simulink model "lab3_ss_srl"  (R2024b)
settings: Solver=ode45  StartTime=0.0  StopTime=sIn.simulation_time  RelTol=1e-3
undefined symbols (not defined in the file or in its folder): daq, DiscIntNeverNeededParam, drv, feedback, filt, gbox, mld, mot, rads2rpm, sens, sIn
libraries: simulink x1
settings Model: Creator=pries  LastModifiedBy=Nihal
settings DataIOCC: SaveOutput=off  SaveTime=off  ReturnWorkspaceOutputs=off

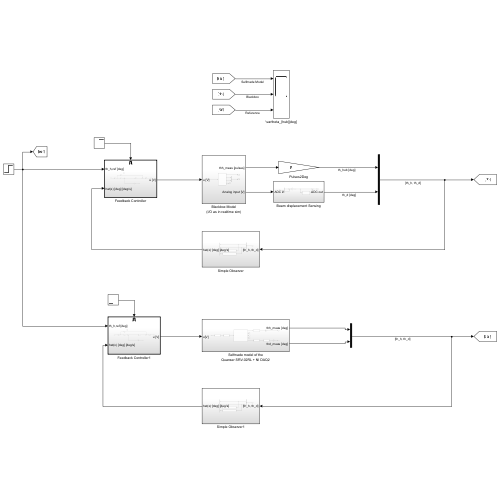
[thumbnail: Simulink's stored preview of the top-level diagram]
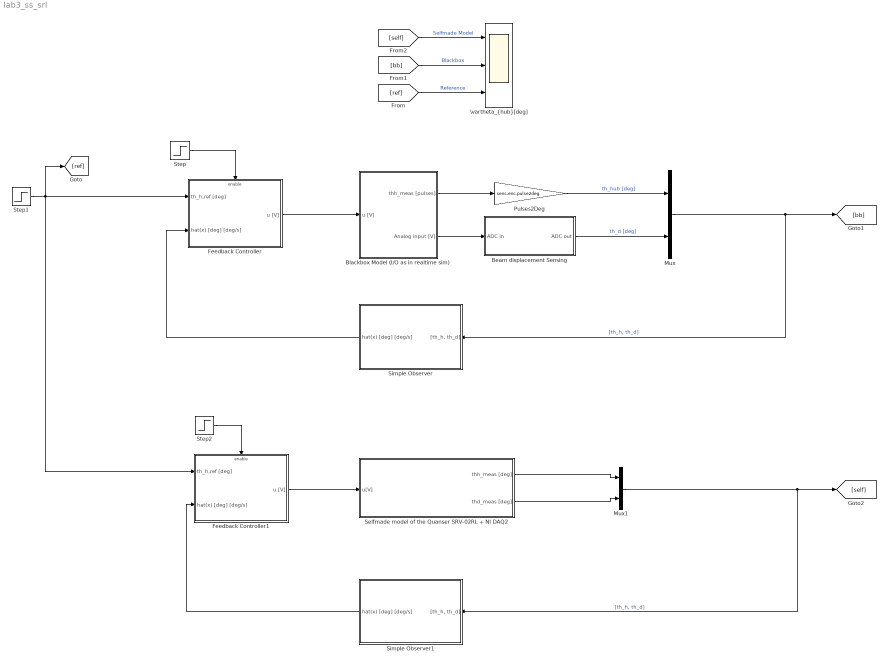
== system lab3_ss_srl ==
  Beam displacement Sensing : Subsystem
  Blackbox Model (I/O as in realtime sim) : Subsystem
  Feedback Controller : Subsystem
  Feedback Controller1 : Subsystem
  Mux : Mux  Inputs=2
  Mux1 : Mux  Inputs=2
  Pulses2Deg : Gain  Gain=sens.enc.pulse2deg
  Selfmade model of the Quanser SRV-02RL + NI DAQ2 : Subsystem
  Simple Observer : Subsystem
  Simple Observer1 : Subsystem
  Step : Step  Time=sIn.t1  SampleTime=0
  Step1 : Step  Time=sIn.t1  After=sIn.position  SampleTime=0
  Step2 : Step  Time=sIn.t1  SampleTime=0
  "\\vartheta_{hub}[deg]" : Scope  NumInputPorts=3
  wires:
  Pulses2Deg/1 -> Mux/1  "th_hub [deg]"
  Mux/1 -> [bb], Simple Observer/1("[th_h, th_d]")  "[th_h, th_d]"
  Simple Observer/1(hat(x) [deg] [deg/s]) -> Feedback Controller/2(hat(x) [deg] [deg/s])
  Blackbox Model (I/O as in realtime sim)/1(thh_meas [pulses]) -> Pulses2Deg/1
  Blackbox Model (I/O as in realtime sim)/2(Analog input [V]) -> Beam displacement Sensing/1(ADC in)
  Beam displacement Sensing/1(ADC out) -> Mux/2  "th_d [deg]"
  Step/1 -> Feedback Controller/Enable
  Feedback Controller/1(u [V]) -> Blackbox Model (I/O as in realtime sim)/1(u [V])
  Step1/1 -> Feedback Controller1/1(th_h,ref [deg]), Feedback Controller/1(th_h,ref [deg]), [ref]
  Simple Observer1/1(hat(x) [deg] [deg/s]) -> Feedback Controller1/2(hat(x) [deg] [deg/s])
  Mux1/1 -> Simple Observer1/1("[th_h, th_d]"), [self]  "[th_h, th_d]"
  [self] -> "\\vartheta_{hub}[deg]"/1  "Selfmade Model"
  [bb] -> "\\vartheta_{hub}[deg]"/2  "Blackbox"
  [ref] -> "\\vartheta_{hub}[deg]"/3  "Reference"
  Feedback Controller1/1(u [V]) -> Selfmade model of the Quanser SRV-02RL + NI DAQ2/1(u[V])
  Step2/1 -> Feedback Controller1/Enable
  Selfmade model of the Quanser SRV-02RL + NI DAQ2/1(thh_meas [deg]) -> Mux1/1
  Selfmade model of the Quanser SRV-02RL + NI DAQ2/2(thd_meas [deg]) -> Mux1/2

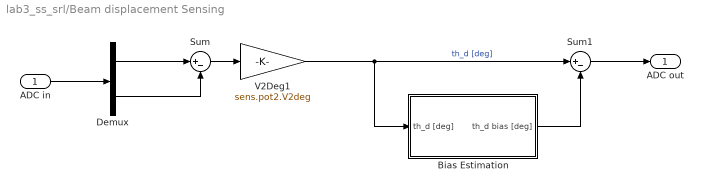
== system lab3_ss_srl/Beam displacement Sensing ==
  ADC in : Inport
  Bias Estimation : Subsystem
  Demux : Demux  Outputs=2
  Sum : Sum  Inputs=|+-
  Sum1 : Sum  Inputs=|+-
  V2Deg1 : Gain  Gain=sens.pot2.V2deg
  ADC out : Outport
  wires:
  Bias Estimation/1(th_d bias [deg]) -> Sum1/2
  ADC in/1 -> Demux/1
  V2Deg1/1 -> Bias Estimation/1(th_d [deg]), Sum1/1  "th_d [deg]"
  Sum/1 -> V2Deg1/1
  Demux/2 -> Sum/2
  Demux/1 -> Sum/1
  Sum1/1 -> ADC out/1

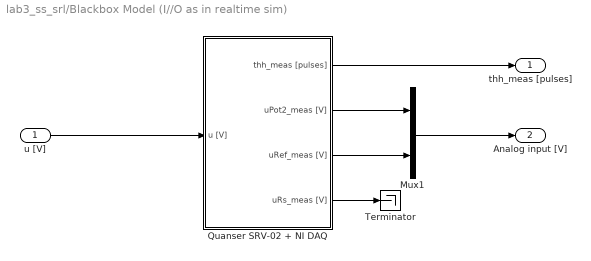
== system lab3_ss_srl/Blackbox Model (I//O as in realtime sim) ==
  u [V] : Inport
  Mux1 : Mux  Inputs=2
  Quanser SRV-02 + NI DAQ : Subsystem  mask(Quanser SRV-02 (with resonant load) + NI DAQ){Ts=0.001, fricType=Coulomb + viscous, lockShaft=off, beamInitPos=10}
      mask prompts: Ts "NI DAQ Sample Time:"; fricType "Friction model"; lockShaft "Lock motor shaft"; beamInitPos "Beam initial position [deg]:"
      mask help: Quanser SRV-02 (with resonant load) + NI DAQ model.
      mask init:
      | %%
      | % Riccardo Antonello (riccardo.antonello@unipd.it)
      | %
      | % April 28, 2020
      | %
      | % Dept. of Information Engineering, University of Padova
      | %
      | 
      | %%  Conversion gains
      | deg2rad = pi/180;                   %   [deg]   -> [rad]
      | rad2deg = 180/pi;                   %   [rad]   -> [deg]
      | 
      | 
      | %%  Sensors data
      | 
      | %   shunt resistor
      | sens.curr.Rs = 0.5;   
      | 
      | %   Hewlett-Packard HEDS-5540#A06 optical encoder
      | sens.enc.ppr = 500*4;                                                   %   pulses per rotation
      | sens.enc.pulse2deg = 360/sens.enc.ppr;                                  %   [pulses] -> [deg]
      | sens.enc.pulse2rad = 2*pi/sens.enc.ppr;                                 %   [pulses] -> [rad]
      | sens.enc.deg2pulse = sens.enc.ppr/360;                                  %   [deg] -> [pulses]
      | sens.enc.rad2pulse = sens.enc.ppr/2/pi;                                 %   [rad] -> [pulses]
      | 
      | %   potentiometer 2 (Spectrol 357-0-0-103) - installed on hub
      | sens.pot2.range.R      = 10e3;                                          %   ohmic value range 
      | sens.pot2.range.V      = 5;                                             %   voltage range
      | sens.pot2.range.th_deg = 340;                                           %   angle range [deg]
      | sens.pot2.range.th     = sens.pot2.range.th_deg * deg2rad;              %   angle range [rad]                           
      | sens.pot2.deg2V        = sens.pot2.range.V / sens.pot2.range.th_deg;    %   sensitivity [V/deg]
      | sens.pot2.rad2V        = sens.pot2.range.V / sens.pot2.range.th;        %   sensitivity [V/rad]
      | sens.pot2.V2deg        = 1/sens.pot2.deg2V;                             %   conversion gain [V] -> [deg]
      | sens.pot2.V2rad        = 1/sens.pot2.rad2V;                             %   conversion gain [V] -> [rad]
      | sens.pot2.noise.var    = 3.5e-7;                                        %   out noise variance [V^2]
      | 
      | 
      | %%  Data acquisition board (daq) data
      | 
      | %   NI PCI-6221 DAC data
      | daq.dac.bits = 16;                                  %   resolution (bits)
      | daq.dac.fs   = 10;                                  %   full scale 
      | daq.dac.q    = 2*daq.dac.fs/(2^daq.dac.bits-1);     %	quantization
      | 
      | %   NI PCI-6221 ADC data
      | daq.adc.bits = 16;                                  %   resolution (bits)
      | daq.adc.fs   = 10;                                  %   full scale (as set in SLDRT Analog Input block)
      | daq.adc.q    = 2*daq.adc.fs/(2^daq.adc.bits-1);     %   quantization   
      | 
      | 
      | %%  Set beam initial position
      | % SRV02Handle = find_system(gcb, ...
      | %     'LookUnderMasks', 'on', ...
      | %     'FindAll', 'on', ...
      | %     'FollowLinks', 'on', ...
      | %     'SearchDepth', '1', ...
      | %     'BlockType', 'ModelReference', ...
      | %     'Name', 'Quanser SRV-02');
      | %
      | % %get_param(SRV02Handle, 'InstanceParameters')
      | % InstanceParams = get_param(SRV02Handle, 'InstanceParameters');
      | % for k = 1:length(InstanceParams)
      | %     if strcmp(InstanceParams(k).Name, 'thb0')
      | %         if lockShaft
      | %             InstanceParams(k).Value = sprintf('%f', beamInitPos);
      | %         else
      | %             InstanceParams(k).Value = sprintf('%f', 0);    
      | %         end
      | %         set_param(SRV02Handle, 'InstanceParameters', InstanceParams);
      | %         break;
      | %     end
      | % end
      | 
      | if lockShaft
      |     thb0 = beamInitPos;
      | else
      |     thb0 = 0;    
      | end
      | 
      | 
      | %%  Mask initialization
      | if lockShaft
      |     
      |     %   find Inport handle
      |     InPortHandle = find_system(gcb, ...
      |         'LookUnderMasks', 'on', ...
      |         'FindAll', 'on', ...
      |         'FollowLinks', 'on', ...
      |         'SearchDepth', '1', ...
      |         'BlockType', 'Inport', ...
      |         'Name', 'u [V]');
      |     
      |     if ~isempty(InPortHandle)
      |     
      |         %   find DAC handle
      |         DACHandle = find_system(gcb, ...
      |             'LookUnderMasks', 'on', ...
      |             'FindAll', 'on', ...
      |             'FollowLinks', 'on', ...
      |             'SearchDepth', '1', ...
      |             'BlockType', 'SubSystem', ...
      |             'Name', 'DAC');  
      | 
      |         %   remove Inport output connection   
      |         InportConn = get_param(InPortHandle, 'PortConnectivity');
      |         delete_line(gcb, InportConn.Position);
      | 
      |         %   remove Inport block
      |         delete_block(InPortHandle);
      | 
      |         %   add Constant block
      |         ConstantHandle = add_block( ...
      |             'simulink/Sources/Constant', [gcb, '/u [V]'], ...
      |             'Position', [20   -37    50   -23], ...
      |             'Value', '0');
      | 
      |         %   connect Constant to DAC block
      |         DACPortHandles = get_param(DACHandle, 'PortHandles');
      |         ConstantPortHandles = get_param(ConstantHandle, 'PortHandles');
      |         add_line(gcb, ConstantPortHandles.Outport(1), DACPortHandles.Inport(1));
      |     
      |     end
      |     
      | else
      |     
      |     %   find Constant handle
      |     ConstantHandle = find_system(gcb, ...
      |         'LookUnderMasks', 'on', ...
      |         'FindAll', 'on', ...
      |         'FollowLinks', 'on', ...
      |         'SearchDepth', '1', ...
      |         'BlockType', 'Constant', ...
      |         'Name', 'u [V]');
      |     
      |     if ~isempty(ConstantHandle)
      |     
      |         %   find DAC handle
      |         DACHandle = find_system(gcb, ...
      |             'LookUnderMasks', 'on', ...
      |             'FindAll', 'on', ...
      |             'FollowLinks', 'on', ...
      |             'SearchDepth', '1', ...
      |             'BlockType', 'SubSystem', ...
      |             'Name', 'DAC');  
      |  
      |         %   remove Constant output connection   
      |         ConstantConn = get_param(ConstantHandle, 'PortConnectivity');
      |         delete_line(gcb, ConstantConn.Position);
      | 
      |         %   remove Inport block
      |         delete_block(ConstantHandle);   
      | 
      |         %   add Inport block
      |         InportHandle = add_block( ...
      |             'simulink/Sources/In1', [gcb, '/u [V]'], ...
      |             'Position', [20   -37    50   -23], ...
      |             'Port', '1');
      | 
      |         %   connect Constant to DAC block
      |         DACPortHandles = get_param(DACHandle, 'PortHandles');
      |         InportPortHandles = get_param(InportHandle, 'PortHandles');
      |         add_line(gcb, InportPortHandles.Outport(1), DACPortHandles.Inport(1));
      |     
      |      end
      |     
      | end
      mask Help:
      | Riccardo Antonello (antonello@dei.unipd.it)
      | 
      | April 28, 2020
      | 
      | Dept. of Information Engineering, University of Padova
      mask TypeOptions fricType: Coulomb + viscous | Karnopp
      mask Callback lockShaft:
      | %   get status of check box
      | lockShaft = get_param(gcb, 'lockShaft');
      | 
      | %   get current value of MaskVisibilities property
      | maskVisibilities = get_param(gcb, 'MaskVisibilities');
      | 
      | %   set visibility of the dialog box element
      | if strcmp(lockShaft, 'on')
      |     maskVisibilities{4} = 'on';
      | else
      |     maskVisibilities{4} = 'off';
      | end
      | 
      | % Set the 'MaskVisibilities' property for each parameter in mask
      | set_param( gcb, 'MaskVisibilities', maskVisibilities);
  Terminator : Terminator
  thh_meas [pulses] : Outport
  Analog input [V] : Outport  Port=2
  wires:
  Quanser SRV-02 + NI DAQ/1(thh_meas [pulses]) -> thh_meas [pulses]/1
  Quanser SRV-02 + NI DAQ/4(uRs_meas [V]) -> Terminator/1
  Mux1/1 -> Analog input [V]/1
  Quanser SRV-02 + NI DAQ/3(uRef_meas [V]) -> Mux1/2
  Quanser SRV-02 + NI DAQ/2(uPot2_meas [V]) -> Mux1/1
  u [V]/1 -> Quanser SRV-02 + NI DAQ/1(u [V])

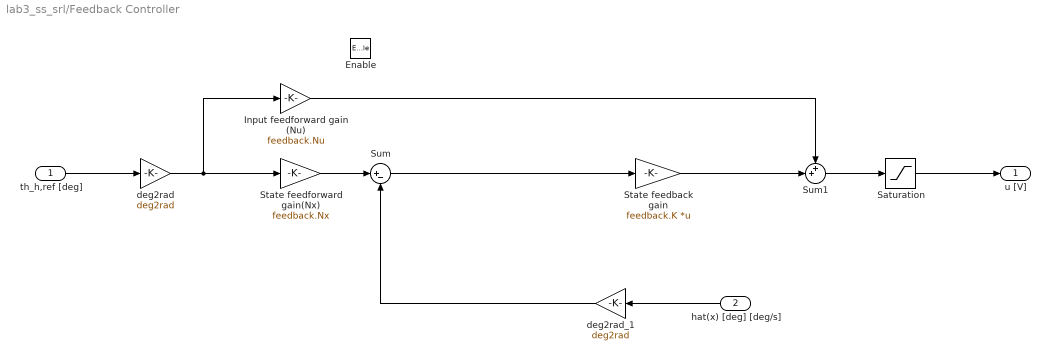
== system lab3_ss_srl/Feedback Controller ==
  th_h,ref [deg] : Inport
  hat(x) [deg] [deg/s] : Inport  Port=2
  Enable : EnablePort
  Input feedforward gain (Nu) : Gain  Gain=feedback.Nu
  Saturation : Saturate  UpperLimit=10  LowerLimit=-10
  State feedback gain : Gain  Gain=feedback.K  Multiplication=Matrix(K*u)
  State feedforward gain(Nx) : Gain  Gain=feedback.Nx
  Sum : Sum  Inputs=|+-
  Sum1 : Sum  Inputs=++|
  deg2rad : Gain  Gain=deg2rad
  deg2rad_1 : Gain  Gain=deg2rad
  u [V] : Outport
  wires:
  deg2rad_1/1 -> Sum/2
  Input feedforward gain (Nu)/1 -> Sum1/1
  State feedback gain/1 -> Sum1/2
  Sum1/1 -> Saturation/1
  Sum/1 -> State feedback gain/1
  Saturation/1 -> u [V]/1
  State feedforward gain(Nx)/1 -> Sum/1
  deg2rad/1 -> State feedforward gain(Nx)/1, Input feedforward gain (Nu)/1
  th_h,ref [deg]/1 -> deg2rad/1
  hat(x) [deg] [deg/s]/1 -> deg2rad_1/1

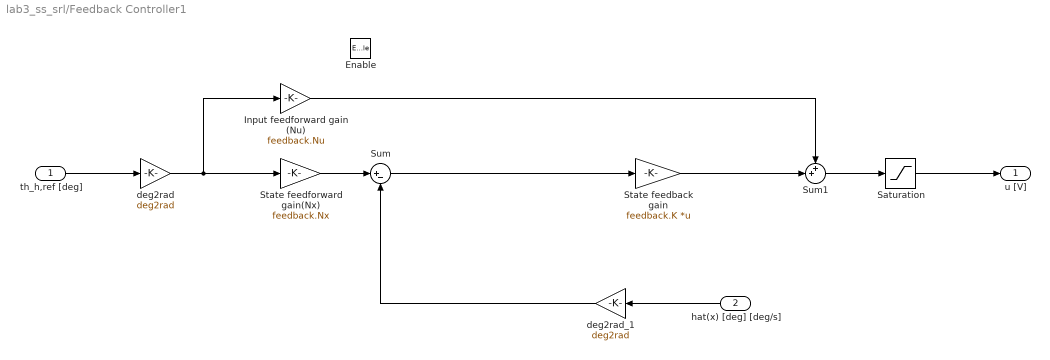
== system lab3_ss_srl/Feedback Controller1 ==
  th_h,ref [deg] : Inport
  hat(x) [deg] [deg/s] : Inport  Port=2
  Enable : EnablePort
  Input feedforward gain (Nu) : Gain  Gain=feedback.Nu
  Saturation : Saturate  UpperLimit=10  LowerLimit=-10
  State feedback gain : Gain  Gain=feedback.K  Multiplication=Matrix(K*u)
  State feedforward gain(Nx) : Gain  Gain=feedback.Nx
  Sum : Sum  Inputs=|+-
  Sum1 : Sum  Inputs=++|
  deg2rad : Gain  Gain=deg2rad
  deg2rad_1 : Gain  Gain=deg2rad
  u [V] : Outport
  wires:
  deg2rad_1/1 -> Sum/2
  Input feedforward gain (Nu)/1 -> Sum1/1
  State feedback gain/1 -> Sum1/2
  Sum1/1 -> Saturation/1
  Sum/1 -> State feedback gain/1
  Saturation/1 -> u [V]/1
  State feedforward gain(Nx)/1 -> Sum/1
  deg2rad/1 -> State feedforward gain(Nx)/1, Input feedforward gain (Nu)/1
  th_h,ref [deg]/1 -> deg2rad/1
  hat(x) [deg] [deg/s]/1 -> deg2rad_1/1

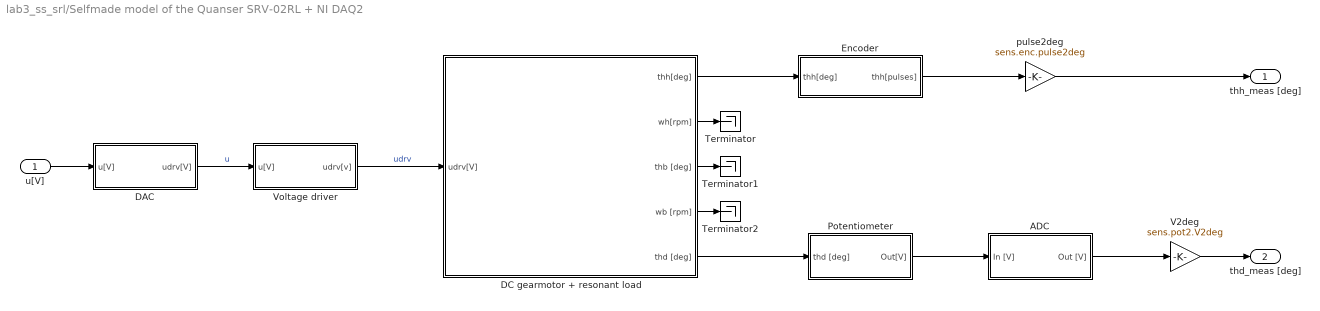
== system lab3_ss_srl/Selfmade model of the Quanser SRV-02RL + NI DAQ2 ==
  u[V] : Inport
  ADC : Subsystem
  DAC : Subsystem
  DC gearmotor + resonant load : Subsystem
  Encoder : Subsystem
  Potentiometer : Subsystem
  Terminator : Terminator
  Terminator1 : Terminator
  Terminator2 : Terminator
  V2deg : Gain  Gain=sens.pot2.V2deg
  Voltage driver : Subsystem
  pulse2deg : Gain  Gain=sens.enc.pulse2deg
  thh_meas [deg] : Outport
  thd_meas [deg] : Outport  Port=2
  wires:
  u[V]/1 -> DAC/1(u[V])
  DAC/1(udrv[V]) -> Voltage driver/1(u[V])  "u"
  Voltage driver/1(udrv[v]) -> DC gearmotor + resonant load/1(udrv[V])  "udrv"
  DC gearmotor + resonant load/1(thh[deg]) -> Encoder/1(thh[deg])
  Encoder/1(thh[pulses]) -> pulse2deg/1
  pulse2deg/1 -> thh_meas [deg]/1
  V2deg/1 -> thd_meas [deg]/1
  DC gearmotor + resonant load/5(thd [deg]) -> Potentiometer/1(thd [deg])
  DC gearmotor + resonant load/4(wb [rpm]) -> Terminator2/1
  DC gearmotor + resonant load/3(thb [deg]) -> Terminator1/1
  DC gearmotor + resonant load/2(wh[rpm]) -> Terminator/1
  Potentiometer/1(Out[V]) -> ADC/1(In [V])
  ADC/1(Out [V]) -> V2deg/1

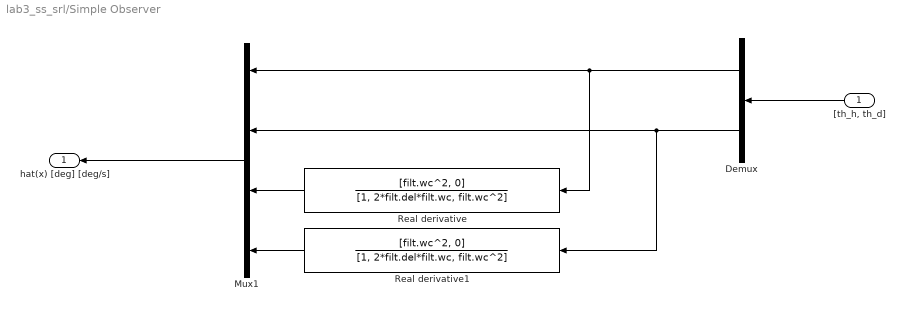
== system lab3_ss_srl/Simple Observer ==
  "[th_h, th_d]" : Inport
  Demux : Demux  Outputs=2
  Mux1 : Mux
  Real derivative : TransferFcn  Numerator=[filt.wc^2, 0]  Denominator=[1, 2*filt.del*filt.wc, filt.wc^2]
  Real derivative1 : TransferFcn  Numerator=[filt.wc^2, 0]  Denominator=[1, 2*filt.del*filt.wc, filt.wc^2]
  hat(x) [deg] [deg/s] : Outport
  wires:
  Demux/1 -> Mux1/1, Real derivative/1
  Mux1/1 -> hat(x) [deg] [deg/s]/1
  "[th_h, th_d]"/1 -> Demux/1
  Real derivative/1 -> Mux1/3
  Demux/2 -> Real derivative1/1, Mux1/2
  Real derivative1/1 -> Mux1/4

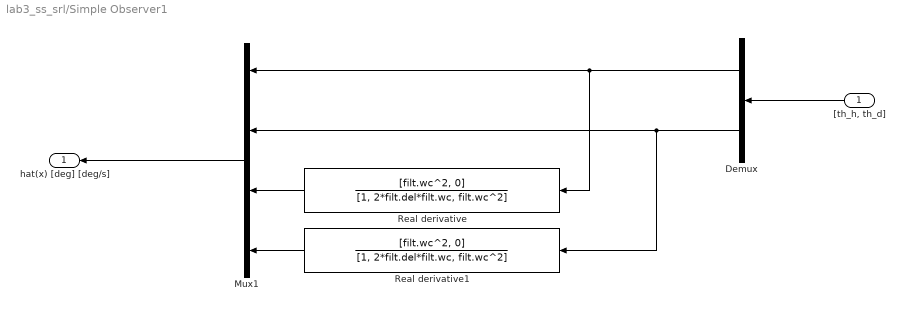
== system lab3_ss_srl/Simple Observer1 ==
  "[th_h, th_d]" : Inport
  Demux : Demux  Outputs=2
  Mux1 : Mux
  Real derivative : TransferFcn  Numerator=[filt.wc^2, 0]  Denominator=[1, 2*filt.del*filt.wc, filt.wc^2]
  Real derivative1 : TransferFcn  Numerator=[filt.wc^2, 0]  Denominator=[1, 2*filt.del*filt.wc, filt.wc^2]
  hat(x) [deg] [deg/s] : Outport
  wires:
  Real derivative1/1 -> Mux1/4
  Demux/2 -> Mux1/2, Real derivative1/1
  Real derivative/1 -> Mux1/3
  "[th_h, th_d]"/1 -> Demux/1
  Mux1/1 -> hat(x) [deg] [deg/s]/1
  Demux/1 -> Real derivative/1, Mux1/1

== system lab3_ss_srl/Beam displacement Sensing/Bias Estimation ==
  th_d [deg] : Inport
  Average : Subsystem
  Clock : Clock
  Interval Test : simulink/Logic and Bit Operations/Interval Test  IntervalClosedRight=on  uplimit=sIn.t1  IntervalClosedLeft=on  lowlimit=sIn.t0  OutDataTypeStr=boolean
  th_d bias [deg] : Outport
  wires:
  Average/1(Out) -> th_d bias [deg]/1
  th_d [deg]/1 -> Average/1(In)
  Interval Test/1 -> Average/Enable
  Clock/1 -> Interval Test/1

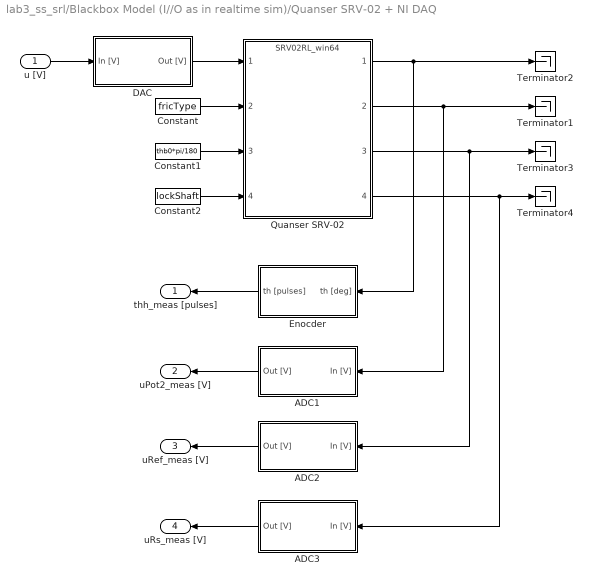
== system lab3_ss_srl/Blackbox Model (I//O as in realtime sim)/Quanser SRV-02 + NI DAQ ==
  u [V] : Inport
  ADC1 : Subsystem
  ADC2 : Subsystem
  ADC3 : Subsystem
  Constant : Constant  Value=fricType
  Constant1 : Constant  Value=thb0*pi/180  SampleTime=Inf
  Constant2 : Constant  Value=lockShaft  SampleTime=Inf
  DAC : Subsystem
  Enocder : Subsystem
  Quanser SRV-02 : ModelReference  ModelNameDialog=SRV02RL_win64.slxp  ModelReferenceVersion=1.76  CopyOfModelProtected=on
  Terminator{1..4} (4 alike) : Terminator
  thh_meas [pulses] : Outport
  uPot2_meas [V] : Outport  Port=2
  uRef_meas [V] : Outport  Port=3
  uRs_meas [V] : Outport  Port=4
  wires:
  ADC2/1(Out [V]) -> uRef_meas [V]/1
  Quanser SRV-02/4 -> Terminator4/1, ADC3/1(In [V])
  Constant2/1 -> Quanser SRV-02/4
  Constant1/1 -> Quanser SRV-02/3
  ADC1/1(Out [V]) -> uPot2_meas [V]/1
  Quanser SRV-02/3 -> Terminator3/1, ADC2/1(In [V])
  Constant/1 -> Quanser SRV-02/2
  Quanser SRV-02/1 -> Enocder/1(th [deg]), Terminator2/1
  Quanser SRV-02/2 -> Terminator1/1, ADC1/1(In [V])
  DAC/1(Out [V]) -> Quanser SRV-02/1
  ADC3/1(Out [V]) -> uRs_meas [V]/1
  Enocder/1(th [pulses]) -> thh_meas [pulses]/1
  u [V]/1 -> DAC/1(In [V])

== system lab3_ss_srl/Selfmade model of the Quanser SRV-02RL + NI DAQ2/ADC ==
  In [V] : Inport
  ADC Sampling : ZeroOrderHold  SampleTime=daq.adc.Ts
  ADC Saturation : Saturate  UpperLimit=2.5  LowerLimit=-2.5
  ADC quantization : Quantizer  QuantizationInterval=daq.adc.q
  Out [V] : Outport
  wires:
  In [V]/1 -> ADC Sampling/1
  ADC Sampling/1 -> ADC quantization/1
  ADC quantization/1 -> ADC Saturation/1
  ADC Saturation/1 -> Out [V]/1

== system lab3_ss_srl/Selfmade model of the Quanser SRV-02RL + NI DAQ2/DAC ==
  u[V] : Inport
  Quantizer : Quantizer  QuantizationInterval=daq.dac.q
  Saturation : Saturate  UpperLimit=10  LowerLimit=-10
  Zero-Order Hold : ZeroOrderHold  SampleTime=1e-3
  udrv[V] : Outport
  wires:
  Zero-Order Hold/1 -> Quantizer/1
  u[V]/1 -> Zero-Order Hold/1
  Quantizer/1 -> Saturation/1
  Saturation/1 -> udrv[V]/1

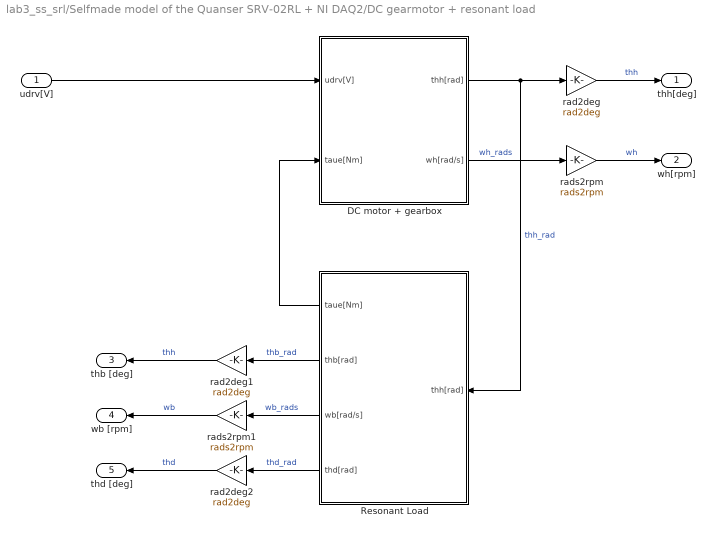
== system lab3_ss_srl/Selfmade model of the Quanser SRV-02RL + NI DAQ2/DC gearmotor + resonant load ==
  udrv[V] : Inport
  DC motor + gearbox : Subsystem
  Resonant Load : Subsystem
  rad2deg : Gain  Gain=rad2deg
  rad2deg1 : Gain  Gain=rad2deg
  rad2deg2 : Gain  Gain=rad2deg
  rads2rpm : Gain  Gain=rads2rpm
  rads2rpm1 : Gain  Gain=rads2rpm
  thh[deg] : Outport
  wh[rpm] : Outport  Port=2
  thb [deg] : Outport  Port=3
  wb [rpm] : Outport  Port=4
  thd [deg] : Outport  Port=5
  wires:
  DC motor + gearbox/1(thh[rad]) -> Resonant Load/1(thh[rad]), rad2deg/1  "thh_rad"
  Resonant Load/2(thb[rad]) -> rad2deg1/1  "thb_rad"
  rad2deg2/1 -> thd [deg]/1  "thd"
  rad2deg/1 -> thh[deg]/1  "thh"
  Resonant Load/4(thd[rad]) -> rad2deg2/1  "thd_rad"
  Resonant Load/1(taue[Nm]) -> DC motor + gearbox/2(taue[Nm])
  rad2deg1/1 -> thb [deg]/1  "thh"
  rads2rpm1/1 -> wb [rpm]/1  "wb"
  Resonant Load/3(wb[rad/s]) -> rads2rpm1/1  "wb_rads"
  DC motor + gearbox/2(wh[rad/s]) -> rads2rpm/1  "wh_rads"
  rads2rpm/1 -> wh[rpm]/1  "wh"
  udrv[V]/1 -> DC motor + gearbox/1(udrv[V])

== system lab3_ss_srl/Selfmade model of the Quanser SRV-02RL + NI DAQ2/Encoder ==
  thh[deg] : Inport
  Gain : Gain  Gain=1/sens.enc.pulse2deg
  Quantizer : Quantizer  QuantizationInterval=sens.enc.pulse2deg
  Zero-Order Hold : ZeroOrderHold  SampleTime=1e-3
  thh[pulses] : Outport
  wires:
  thh[deg]/1 -> Zero-Order Hold/1
  Gain/1 -> thh[pulses]/1
  Quantizer/1 -> Gain/1
  Zero-Order Hold/1 -> Quantizer/1

== system lab3_ss_srl/Selfmade model of the Quanser SRV-02RL + NI DAQ2/Potentiometer ==
  thd [deg] : Inport
  Sensor output noise [V] : RandomNumber  Variance=sens.pot2.noise.var  SampleTime=daq.adc.Ts
  Sum : Sum  Inputs=|++
  deg2V : Gain  Gain=sens.pot2.deg2V
  Out[V] : Outport
  wires:
  thd [deg]/1 -> deg2V/1
  deg2V/1 -> Sum/1
  Sensor output noise [V]/1 -> Sum/2
  Sum/1 -> Out[V]/1

== system lab3_ss_srl/Selfmade model of the Quanser SRV-02RL + NI DAQ2/Voltage driver ==
  u[V] : Inport
  Saturation : Saturate  UpperLimit=12  LowerLimit=-12
  Transfer Fcn : TransferFcn  Numerator=[drv.dcgain]  Denominator=[drv.Tc 1]
  udrv[v] : Outport
  wires:
  u[V]/1 -> Transfer Fcn/1
  Transfer Fcn/1 -> Saturation/1
  Saturation/1 -> udrv[v]/1

== system lab3_ss_srl/Beam displacement Sensing/Bias Estimation/Average ==
  In : Inport
  Enable : EnablePort
  Discrete-Time Integrator : DiscreteIntegrator  gainval=1/(sIn.t1-sIn.t0)  SampleTime=-1  ICPrevOutput=DiscIntNeverNeededParam  ICPrevScaledInput=DiscIntNeverNeededParam
  Out : Outport
  wires:
  Discrete-Time Integrator/1 -> Out/1
  In/1 -> Discrete-Time Integrator/1

== system lab3_ss_srl/Blackbox Model (I//O as in realtime sim)/Quanser SRV-02 + NI DAQ/ADC1 ==
  In [V] : Inport
  ADC quantization : Quantizer  QuantizationInterval=daq.adc.q
  ADC sampling : ZeroOrderHold  SampleTime=Ts
  ADC saturation : Saturate  UpperLimit=daq.adc.fs  LowerLimit=-daq.adc.fs
  Out [V] : Outport
  wires:
  ADC quantization/1 -> ADC saturation/1
  In [V]/1 -> ADC sampling/1
  ADC sampling/1 -> ADC quantization/1
  ADC saturation/1 -> Out [V]/1

== system lab3_ss_srl/Blackbox Model (I//O as in realtime sim)/Quanser SRV-02 + NI DAQ/ADC2 ==
  In [V] : Inport
  ADC quantization : Quantizer  QuantizationInterval=daq.adc.q
  ADC sampling : ZeroOrderHold  SampleTime=Ts
  ADC saturation : Saturate  UpperLimit=daq.adc.fs  LowerLimit=-daq.adc.fs
  Out [V] : Outport
  wires:
  ADC saturation/1 -> Out [V]/1
  ADC sampling/1 -> ADC quantization/1
  In [V]/1 -> ADC sampling/1
  ADC quantization/1 -> ADC saturation/1

== system lab3_ss_srl/Blackbox Model (I//O as in realtime sim)/Quanser SRV-02 + NI DAQ/ADC3 ==
  In [V] : Inport
  Quantizer : Quantizer  QuantizationInterval=daq.adc.q
  Saturation : Saturate  UpperLimit=daq.adc.fs  LowerLimit=-daq.adc.fs
  Zero-Order Hold : ZeroOrderHold  SampleTime=Ts
  Out [V] : Outport
  wires:
  Zero-Order Hold/1 -> Quantizer/1
  Quantizer/1 -> Saturation/1
  In [V]/1 -> Zero-Order Hold/1
  Saturation/1 -> Out [V]/1

== system lab3_ss_srl/Blackbox Model (I//O as in realtime sim)/Quanser SRV-02 + NI DAQ/DAC ==
  In [V] : Inport
  Quantizer : Quantizer  QuantizationInterval=daq.dac.q
  Saturation : Saturate  UpperLimit=daq.dac.fs  LowerLimit=-daq.dac.fs
  Zero-Order Hold : ZeroOrderHold  SampleTime=Ts
  Out [V] : Outport
  wires:
  Saturation/1 -> Out [V]/1
  Zero-Order Hold/1 -> Quantizer/1
  In [V]/1 -> Zero-Order Hold/1
  Quantizer/1 -> Saturation/1

== system lab3_ss_srl/Blackbox Model (I//O as in realtime sim)/Quanser SRV-02 + NI DAQ/Enocder ==
  th [deg] : Inport
  Quantizer : Quantizer  QuantizationInterval=sens.enc.pulse2deg
  Zero-Order Hold : ZeroOrderHold  SampleTime=Ts
  deg2pulse : Gain  Gain=sens.enc.deg2pulse
  th [pulses] : Outport
  wires:
  deg2pulse/1 -> th [pulses]/1
  Zero-Order Hold/1 -> Quantizer/1
  th [deg]/1 -> Zero-Order Hold/1
  Quantizer/1 -> deg2pulse/1

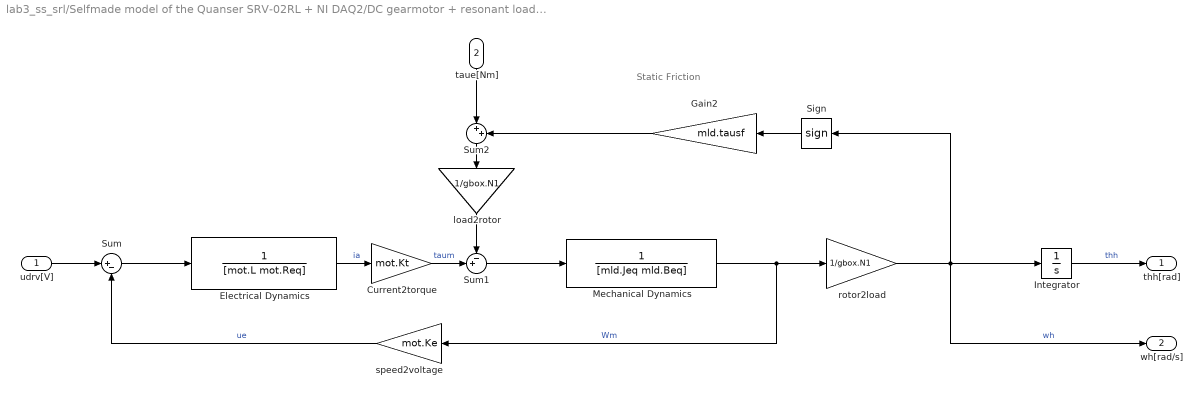
== system lab3_ss_srl/Selfmade model of the Quanser SRV-02RL + NI DAQ2/DC gearmotor + resonant load/DC motor + gearbox ==
  note: Static Friction
  udrv[V] : Inport
  taue[Nm] : Inport  Port=2
  Current2torque : Gain  Gain=mot.Kt
  Electrical Dynamics : TransferFcn  Denominator=[mot.L mot.Req]
  Gain2 : Gain  Gain=mld.tausf
  Integrator : Integrator
  Mechanical Dynamics : TransferFcn  Denominator=[mld.Jeq mld.Beq]
  Sign : Signum  ZeroCross=off
  Sum : Sum  Inputs=|+-
  Sum1 : Sum  Inputs=-+|
  Sum2 : Sum  Inputs=|++
  load2rotor : Gain  Gain=1/gbox.N1
  rotor2load : Gain  Gain=1/gbox.N1
  speed2voltage : Gain  Gain=mot.Ke
  thh[rad] : Outport
  wh[rad/s] : Outport  Port=2
  wires:
  udrv[V]/1 -> Sum/1
  Sum/1 -> Electrical Dynamics/1
  Electrical Dynamics/1 -> Current2torque/1  "ia"
  load2rotor/1 -> Sum1/1
  Sign/1 -> Gain2/1
  Mechanical Dynamics/1 -> speed2voltage/1, rotor2load/1  "Wm"
  rotor2load/1 -> wh[rad/s]/1, Sign/1, Integrator/1  "wh"
  Sum1/1 -> Mechanical Dynamics/1
  Current2torque/1 -> Sum1/2  "taum"
  speed2voltage/1 -> Sum/2  "ue"
  Integrator/1 -> thh[rad]/1  "thh"
  taue[Nm]/1 -> Sum2/1
  Sum2/1 -> load2rotor/1
  Gain2/1 -> Sum2/2

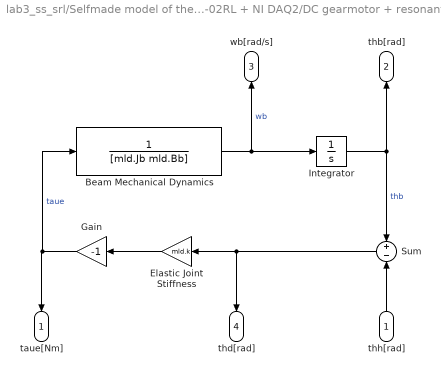
== system lab3_ss_srl/Selfmade model of the Quanser SRV-02RL + NI DAQ2/DC gearmotor + resonant load/Resonant Load ==
  thh[rad] : Inport
  Beam Mechanical Dynamics : TransferFcn  Denominator=[mld.Jb mld.Bb]
  Elastic Joint Stiffness : Gain  Gain=mld.k
  Gain : Gain  Gain=-1
  Integrator : Integrator
  Sum : Sum  Inputs=+|-
  taue[Nm] : Outport
  thb[rad] : Outport  Port=2
  wb[rad/s] : Outport  Port=3
  thd[rad] : Outport  Port=4
  wires:
  thh[rad]/1 -> Sum/2
  Integrator/1 -> Sum/1, thb[rad]/1  "thb"
  Sum/1 -> thd[rad]/1, Elastic Joint Stiffness/1
  Elastic Joint Stiffness/1 -> Gain/1
  Gain/1 -> Beam Mechanical Dynamics/1, taue[Nm]/1  "taue"
  Beam Mechanical Dynamics/1 -> wb[rad/s]/1, Integrator/1  "wb"
